simulink model "pd"  (R2018a)
settings: Solver=VariableStepAuto  StartTime=0.0  StopTime=10.0  RelTol=1e-3
settings Model: Creator=hp  LastModifiedBy=hp

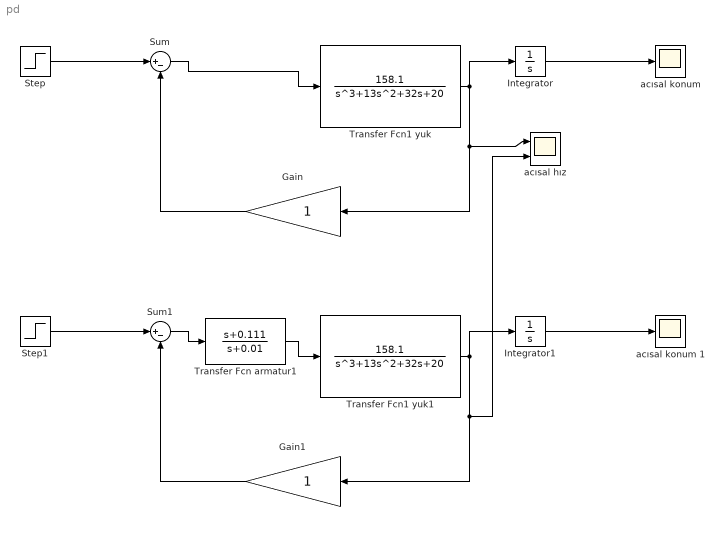
== system pd ==
  Gain : Gain
  Gain1 : Gain
  Integrator : Integrator
  Integrator1 : Integrator
  Step : Step  SampleTime=0
  Step1 : Step  SampleTime=0
  Sum : Sum  Inputs=|+-
  Sum1 : Sum  Inputs=|+-
  Transfer Fcn armatur1 : TransferFcn  Numerator=[1 0.111]  Denominator=[1 0.01]
  Transfer Fcn1 yuk : TransferFcn  Numerator=[158.1]  Denominator=[1 13 32 20]
  Transfer Fcn1 yuk1 : TransferFcn  Numerator=[158.1]  Denominator=[1 13 32 20]
  acısal hız : Scope  NumInputPorts=2
  "acısal konum " : Scope
  acısal konum 1 : Scope
  wires:
  Step/1 -> Sum/1
  Sum/1 -> Transfer Fcn1 yuk/1
  Transfer Fcn1 yuk/1 -> Integrator/1, Gain/1, acısal hız/1
  Integrator/1 -> "acısal konum "/1
  Gain/1 -> Sum/2
  Gain1/1 -> Sum1/2
  Step1/1 -> Sum1/1
  Integrator1/1 -> acısal konum 1/1
  Transfer Fcn1 yuk1/1 -> Integrator1/1, acısal hız/2, Gain1/1
  Transfer Fcn armatur1/1 -> Transfer Fcn1 yuk1/1
  Sum1/1 -> Transfer Fcn armatur1/1
